simulink model "VHF_central_unit"  (R2024a)
settings: Solver=FixedStepDiscrete  StartTime=0.0  StopTime=10.0  FixedStep=0.001  RelTol=1e-3  EnableMultiTasking=on
PreLoadFcn:
  | try
  | MDL_install;
  | catch
  | end
InitFcn:
  | EcoCoder_PreCheckLic();
undefined symbols (not defined in the file or in its folder): C_ROTSPD_ZERO, C_SOC_ZERO, h, km, s, V
libraries: CoderSF_BSW_Libs x222, SF_CanService_Libs x16, CoderSF_ADC2Volt_Libs x6, CoderSF_6AxisMEMS_Libs x6, canmsglib x3, EV_ASWLibs x2, simulink x2, Chassis_stability_controllers x1, CoderSF_KeyCycle_Libs x1
(part 3 of 4)

== system VHF_central_unit/ASW_ReadCAN/Read BMS messages/Subsystem ==
  In1 : Inport
  Bus Creator1 : BusCreator  Inputs=4
  Bus Creator2 : BusCreator  Inputs=4
  Bus Selector : BusSelector  OutputSignals=BMS_OperationStatus.BMSBattPackVoltage,BMS_OperationStatus.BMSBattOCV,BMS_OperationStatus.BMSBattPackCurrent,BMS_OperationStatus.BMSPackMaxDischargeCurrent,BMS_OperationStatus.BMSPackMaxChargeCurrent,BMS_StateOfStatus.BMSStateOfCharge,BMS_StateOfStatus.BMSStateOfHealth,BMS_StateOfStatus.BMSStateOfEnergy,BMS_StateOfStatus.BMSBattStoragedEnergy,BMS_StateOfStatus.BMSBattTemperature,BMS_CellVoltage1to8.BMSCellVoltage1,BMS_CellVoltage1to8.BMSCellVoltage2,BMS_CellVoltage1to8.BMSCellVoltage3,BMS_CellVoltage1to8.BMSCellVoltage4,BMS_CellVoltage1to8.BMSCellVoltage5,BMS_CellVoltage1to8.BMSCellVoltage6,BMS_CellVoltage1to8.BMSCellVoltage7,BMS_CellVoltage1to8.BMSCellVoltage8,BMS_CellVoltage9to16.BMSCellVoltage9,BMS_CellVoltage9to16.BMSCellVoltage10,BMS_CellVoltage9to16.BMSCellVoltage11,BMS_CellVoltage9to16.BMSCellVoltage12,BMS_CellVoltage9to16.BMSCellVoltage13,BMS_CellVoltage9to16.BMSCellVoltage14,BMS_CellVoltage9to16.BMSCellVoltage15,BMS_CellVoltage9to16.BMSCellVoltage16  OutputAsBus=on
  Bus Selector1 : BusSelector  OutputSignals=BMS_OperationStatus.signal1,BMS_StateOfStatus.signal1,BMS_CellVoltage1to8.signal1,BMS_CellVoltage9to16.signal1
  Bus Selector2 : BusSelector  OutputSignals=BMS_OperationStatus.signal2,BMS_StateOfStatus.signal2,BMS_CellVoltage1to8.signal2,BMS_CellVoltage9to16.signal2
  Data Type Conversion{,1..7} (8 alike) : DataTypeConversion  SaturateOnIntegerOverflow=off  RndMeth=Floor
  BMSmsgs : Outport
  MsgAvailable : Outport  Port=2
  MsgCount : Outport  Port=3
  wires:
  Bus Selector/1 -> BMSmsgs/1  "BMSmsgs"
  Bus Selector1/1 -> Data Type Conversion/1  "<signal1>"
  Bus Selector1/2 -> Data Type Conversion1/1  "<signal1>"
  Bus Selector1/3 -> Data Type Conversion2/1  "<signal1>"
  Bus Selector1/4 -> Data Type Conversion3/1  "<signal1>"
  Data Type Conversion/1 -> Bus Creator1/1  "MsgAvailable_OperationStatus"
  Data Type Conversion1/1 -> Bus Creator1/2  "MsgAvailable_StateOfStatus"
  Data Type Conversion2/1 -> Bus Creator1/3  "MsgAvailable_CellVoltage1to8"
  Data Type Conversion3/1 -> Bus Creator1/4  "MsgAvailable_CellVoltage9to16"
  Data Type Conversion7/1 -> Bus Creator2/4  "MsgCount_CellVoltage9to16"
  Data Type Conversion4/1 -> Bus Creator2/1  "MsgCount_OperationStatus"
  Bus Selector2/3 -> Data Type Conversion6/1  "<signal2>"
  Data Type Conversion6/1 -> Bus Creator2/3  "MsgCount_CellVoltage1to8"
  Bus Selector2/2 -> Data Type Conversion5/1  "<signal2>"
  Bus Selector2/4 -> Data Type Conversion7/1  "<signal2>"
  Data Type Conversion5/1 -> Bus Creator2/2  "MsgCount_StateOfStatus"
  Bus Selector2/1 -> Data Type Conversion4/1  "<signal2>"
  In1/1 -> Bus Selector2/1, Bus Selector1/1, Bus Selector/1
  Bus Creator1/1 -> MsgAvailable/1  "MsgAvailable"
  Bus Creator2/1 -> MsgCount/1  "MsgCount"

== system VHF_central_unit/ASW_ReadCAN/Read CCU messages/Subsystem ==
  In1 : Inport
  Bus Creator1 : BusCreator  Inputs=2
  Bus Creator2 : BusCreator  Inputs=2
  Bus Selector : BusSelector  OutputSignals=CCU_Status_VCU.CCUDccOutVoltage,CCU_Status_VCU.CCUDccOutCurrent,CCU_Status_VCU.CCUInputCurrent,CCU_Status_VCU.CCUControlMode,CCU_Status_VCU.CCURegenerateMode,CCU_Status_VCU.CCUFaultControl,CCU_Status_VCU.CCUUnderBattVolt,CCU_Status_VCU.CCUOverBattVolt,CCU_Status_VCU.CCUOverInd1Curr,CCU_Status_VCU.CCUOverInd2Curr,CCU_Status_VCU.CCUOverInd3Curr,CCU_Status_VCU.CCULeg1Failure,CCU_Status_VCU.CCULeg2Failure,CCU_Status_VCU.CCULeg3Failure,CCU_Status_VCU.CCUOverOutVolt,CCU_InductorStatus.CCUInductor1Curr,CCU_InductorStatus.CCUInductor2Curr,CCU_InductorStatus.CCUInductor3Curr  OutputAsBus=on
  Bus Selector1 : BusSelector  OutputSignals=CCU_Status_VCU.signal1,CCU_InductorStatus.signal1
  Bus Selector2 : BusSelector  OutputSignals=CCU_Status_VCU.signal2,CCU_InductorStatus.signal2
  Data Type Conversion{,1,4..5} (4 alike) : DataTypeConversion  SaturateOnIntegerOverflow=off  RndMeth=Floor
  CCUmsgs : Outport
  MsgAvailable : Outport  Port=2
  MsgCount : Outport  Port=3
  wires:
  Bus Selector/1 -> CCUmsgs/1  "CCUmsgs"
  Bus Selector1/1 -> Data Type Conversion/1  "<signal1>"
  Bus Selector1/2 -> Data Type Conversion1/1  "<signal1>"
  Data Type Conversion/1 -> Bus Creator1/1  "MsgAvailable_CCU_Status_VCU"
  Data Type Conversion1/1 -> Bus Creator1/2  "MsgAvailable_CCU_InductorStatus"
  Data Type Conversion4/1 -> Bus Creator2/1  "MsgCount_CCU_Status_VCU"
  Bus Selector2/2 -> Data Type Conversion5/1  "<signal2>"
  Data Type Conversion5/1 -> Bus Creator2/2  "MsgCount_CCU_InductorStatus"
  Bus Selector2/1 -> Data Type Conversion4/1  "<signal2>"
  In1/1 -> Bus Selector2/1, Bus Selector1/1, Bus Selector/1
  Bus Creator1/1 -> MsgAvailable/1  "MsgAvailable"
  Bus Creator2/1 -> MsgCount/1  "MsgCount"

== system VHF_central_unit/ASW_ReadCAN/Read GeneratorSystem messages/Subsystem ==
  In1 : Inport
  Bus Creator1 : BusCreator  Inputs=2
  Bus Creator2 : BusCreator  Inputs=2
  Bus Selector : BusSelector  OutputSignals=SCG_Status_VCU.GenSysDccOutVoltage,SCG_Status_VCU.GenSysDccOutCurrent,SCG_Status_VCU.GenSysGenVoltage,SCG_Status_VCU.GenSysGenCurrent,SCG_Status_VCU.GenSysControlMode,SCG_Status_VCU.GenSysAcRelayStatus,SCG_Status_VCU.GenSysLinkPosRelay,SCG_Status_VCU.GenSysFaultControl,SCG_Status_VCU.GenSysOverOutVolt,SCG_Status_VCU.GenSysOverInd1Curr,SCG_Status_VCU.GenSysOverInd2Curr,SCG_Status_VCU.GenSysOverInd3Curr,SCG_Status_VCU.GenSysLeg1Failure,SCG_Status_VCU.GenSysLeg2Failure,SCG_Status_VCU.GenSysLeg3Failure,SCG_ICE_Status.GenSysMotorTorque,SCG_ICE_Status.GenSysMotorSpeed,SCG_ICE_Status.GenSysThrottle  OutputAsBus=on
  Bus Selector1 : BusSelector  OutputSignals=SCG_Status_VCU.signal1,SCG_ICE_Status.signal1
  Bus Selector2 : BusSelector  OutputSignals=SCG_Status_VCU.signal2,SCG_ICE_Status.signal2
  Data Type Conversion{,1,4..5} (4 alike) : DataTypeConversion  SaturateOnIntegerOverflow=off  RndMeth=Floor
  SCGmsgs : Outport
  MsgAvailable : Outport  Port=2
  MsgCount : Outport  Port=3
  wires:
  Bus Selector/1 -> SCGmsgs/1  "SCGmsgs"
  Bus Selector1/1 -> Data Type Conversion/1  "<signal1>"
  Bus Selector1/2 -> Data Type Conversion1/1  "<signal1>"
  Data Type Conversion/1 -> Bus Creator1/1  "MsgAvailable_SCG_Status_VCU"
  Data Type Conversion1/1 -> Bus Creator1/2  "MsgAvailable_SCG_ICE_Status"
  Data Type Conversion4/1 -> Bus Creator2/1  "MsgCount_SCG_Status_VCU"
  Bus Selector2/2 -> Data Type Conversion5/1  "<signal2>"
  Data Type Conversion5/1 -> Bus Creator2/2  "MsgCount_SCG_ICE_Status"
  Bus Selector2/1 -> Data Type Conversion4/1  "<signal2>"
  In1/1 -> Bus Selector2/1, Bus Selector1/1, Bus Selector/1
  Bus Creator1/1 -> MsgAvailable/1  "MsgAvailable"
  Bus Creator2/1 -> MsgCount/1  "MsgCount"

== system VHF_central_unit/ASW_ReadCAN/Read Motor1 messages/Subsystem ==
  In1 : Inport
  Bus Creator1 : BusCreator  Inputs=2
  Bus Creator2 : BusCreator  Inputs=2
  Bus Selector : BusSelector  OutputSignals=Motor1_RUN_STATUS.Motor1Run_direction,Motor1_RUN_STATUS.Motor1Running_mode,Motor1_RUN_STATUS.Motor1Motor_Speed,Motor1_RUN_STATUS.Motor1Fault_Code,Motor1_RUN_STATUS.Motor1ConsumptionMode,Motor1_RUN_STATUS.Motor1SubtotalMileage,Motor1_ELEC_STATUS.Motor1DC_LinkVoltage,Motor1_ELEC_STATUS.Motor1DC_LinkCurrent  OutputAsBus=on
  Bus Selector1 : BusSelector  OutputSignals=Motor1_RUN_STATUS.signal1,Motor1_ELEC_STATUS.signal1
  Bus Selector2 : BusSelector  OutputSignals=Motor1_RUN_STATUS.signal2,Motor1_ELEC_STATUS.signal2
  Data Type Conversion{,1,4..5} (4 alike) : DataTypeConversion  SaturateOnIntegerOverflow=off  RndMeth=Floor
  Motor1msgs : Outport
  MsgAvailable : Outport  Port=2
  MsgCount : Outport  Port=3
  wires:
  Bus Selector/1 -> Motor1msgs/1  "Motor1msgs"
  Bus Selector1/1 -> Data Type Conversion/1  "<signal1>"
  Bus Selector1/2 -> Data Type Conversion1/1  "<signal1>"
  Data Type Conversion/1 -> Bus Creator1/1  "MsgAvailable_RUN_STATUS"
  Data Type Conversion1/1 -> Bus Creator1/2  "MsgAvailable_ELEC_STATUS"
  Data Type Conversion4/1 -> Bus Creator2/1  "MsgCount_RUN_STATUS"
  Bus Selector2/2 -> Data Type Conversion5/1  "<signal2>"
  Data Type Conversion5/1 -> Bus Creator2/2  "MsgCount_ELEC_STATUS"
  Bus Selector2/1 -> Data Type Conversion4/1  "<signal2>"
  In1/1 -> Bus Selector2/1, Bus Selector1/1, Bus Selector/1
  Bus Creator1/1 -> MsgAvailable/1  "MsgAvailable"
  Bus Creator2/1 -> MsgCount/1  "MsgCount"

== system VHF_central_unit/ASW_ReadCAN/Read Motor2 messages/Subsystem ==
  In1 : Inport
  Bus Creator1 : BusCreator  Inputs=2
  Bus Creator2 : BusCreator  Inputs=2
  Bus Selector : BusSelector  OutputSignals=Motor2_RUN_STATUS.Motor2Run_direction,Motor2_RUN_STATUS.Motor2Running_mode,Motor2_RUN_STATUS.Motor2Motor_Speed,Motor2_RUN_STATUS.Motor2Fault_Code,Motor2_RUN_STATUS.Motor2ConsumptionMode,Motor2_RUN_STATUS.Motor2SubtotalMileage,Motor2_ELEC_STATUS.Motor2DC_LinkVoltage,Motor2_ELEC_STATUS.Motor2DC_LinkCurrent  OutputAsBus=on
  Bus Selector1 : BusSelector  OutputSignals=Motor2_RUN_STATUS.signal1,Motor2_ELEC_STATUS.signal1
  Bus Selector2 : BusSelector  OutputSignals=Motor2_RUN_STATUS.signal2,Motor2_ELEC_STATUS.signal2
  Data Type Conversion{,1,4..5} (4 alike) : DataTypeConversion  SaturateOnIntegerOverflow=off  RndMeth=Floor
  Motor2msgs : Outport
  MsgAvailable : Outport  Port=2
  MsgCount : Outport  Port=3
  wires:
  Bus Selector/1 -> Motor2msgs/1  "Motor2msgs"
  Bus Selector1/1 -> Data Type Conversion/1  "<signal1>"
  Bus Selector1/2 -> Data Type Conversion1/1  "<signal1>"
  Data Type Conversion/1 -> Bus Creator1/1  "MsgAvailable_RUN_STATUS"
  Data Type Conversion1/1 -> Bus Creator1/2  "MsgAvailable_ELEC_STATUS"
  Data Type Conversion4/1 -> Bus Creator2/1  "MsgCount_RUN_STATUS"
  Bus Selector2/2 -> Data Type Conversion5/1  "<signal2>"
  Data Type Conversion5/1 -> Bus Creator2/2  "MsgCount_ELEC_STATUS"
  Bus Selector2/1 -> Data Type Conversion4/1  "<signal2>"
  In1/1 -> Bus Selector2/1, Bus Selector1/1, Bus Selector/1
  Bus Creator1/1 -> MsgAvailable/1  "MsgAvailable"
  Bus Creator2/1 -> MsgCount/1  "MsgCount"

== system VHF_central_unit/ASW_SensorInputs/02 vehicle motion request/01 driver torque demand ==
  sigInDrvPedacc_pct1 : Inport
  f : TriggerPort  TriggerType=function-call  VariantControl=(inherit)
  Switch : Switch  Criteria=u2 ~= 0  SaturateOnIntegerOverflow=off  InputSameDT=off
  ecocoder_calibration : CoderSF_BSW_Libs/Calibration & Measurement/Read Calibration  variable_name=vehDrv_flgCal_val  variable_value=0  variable_type=boolean  variable_min=[]  variable_max=[]  unitStr=""  descStr=""
      settings: AttributesFormatString=value:%<variable_value> type:%<variable_type> max:%<variable_max> Min:%<variable_min>
  ecocoder_calibration1 : CoderSF_BSW_Libs/Calibration & Measurement/Read Calibration  variable_name=vehDrv_linspd_val  variable_value=0  variable_type=single  variable_min=[]  variable_max=[]  unitStr=km/h  descStr=""
      settings: AttributesFormatString=value:%<variable_value> type:%<variable_type> max:%<variable_max> Min:%<variable_min>
  ecocoder_calibration2 : CoderSF_BSW_Libs/Calibration & Measurement/Read Calibration  variable_name=vehDrv_pct_val  variable_value=0  variable_type=single  variable_min=[]  variable_max=[]  unitStr=""  descStr=""
      settings: AttributesFormatString=value:%<variable_value> type:%<variable_type> max:%<variable_max> Min:%<variable_min>
  ecocoder_measurement : CoderSF_BSW_Libs/Calibration & Measurement/Write and Read Measurement  variable_name=vehDrv_linspd  variable_value=0  variable_type=single  numD=1  unitStr=km/h  descStr=""
      settings: AttributesFormatString=value:%<variable_value> type:%<variable_type>
  ecocoder_measurement1 : CoderSF_BSW_Libs/Calibration & Measurement/Write and Read Measurement  variable_name=vehDrv_pct  variable_value=0  variable_type=single  numD=1  unitStr=""  descStr=""
      settings: AttributesFormatString=value:%<variable_value> type:%<variable_type>
  ecocoder_measurement2 : CoderSF_BSW_Libs/Calibration & Measurement/Write and Read Measurement  variable_name=vehDrv_trqReq  variable_value=0  variable_type=single  numD=1  unitStr=Nm  descStr=""
      settings: AttributesFormatString=value:%<variable_value> type:%<variable_type>
  vehDrv_trqEcoTracMax_map : CoderSF_BSW_Libs/Calibration & Measurement/2-D Lookup Table  nam=vehDrv_trqEcoTracMax  breakpoint1_type=single  breakpoint1_data=[0 0.1 0.2 0.3 0.4 0.5 0.6 0.7 0.8 0.9 0.95 1]  breakpoint2_type=single  breakpoint2_data="[0 2 3 10  20 30 40 50 60 70 80 90 95 100 115 120]"  table_type=single  table_data=|
      | [0 0 0 0 0 0 0 0 0 0 0 0 0 0 0 0 ;
      | 0 200 441 439 437 435 433 431 429 427 425 423 421 419 417 415 ;
      | 0 202 461 459 457 455 453 451 449 447 445 443 441 439 437 435 ;
      | 0 204 565 560 555 550 545 540 535 530 525 520 515 510 505 500 ;
      | 0 206 614 611 608 605 602 599 596 593 590 587 584 581 578 575 ;
      | 0 208 678 677 676 675 674 673 672 671 670 669 668 667 666 665 ;
      | 0 210 784 781 778 775 772 769 766 763 760 757 754 751 748 745 ;
      | 0 212 956 954 952 950 948 946 944 942 940 938 936 934 932 930 ;
      | 0 214 1078 1077 1076 1075 1074 1073 1072 1071 1070 1069 1068 1067 1066 1065 ;
      | 0 216 1376 1374 1372 1370 1368 1366 1364 1362 1360 1358 1356 1354 1352 1350 ;
      | 0 218 1576 1574 1572 1570 1568 1566 1564 1562 1560 1558 1556 1554 1552 1550 ;
      | 0 220 1900 1900 1900 1900 1900 1900 1900 1900 1900 1900 1900 1900 1900 1900 ]
  vehDrv_trqReq1 : Outport
  wires:
  vehDrv_trqEcoTracMax_map/1 -> ecocoder_measurement2/1
  ecocoder_calibration1/1 -> ecocoder_measurement/1
  sigInDrvPedacc_pct1/1 -> Switch/3
  Switch/1 -> ecocoder_measurement1/1
  ecocoder_calibration/1 -> Switch/2
  ecocoder_calibration2/1 -> Switch/1
  ecocoder_measurement/1 -> vehDrv_trqEcoTracMax_map/2  "vehDrv_linspd"
  ecocoder_measurement1/1 -> vehDrv_trqEcoTracMax_map/1  "vehDrv_pct"
  ecocoder_measurement2/1 -> vehDrv_trqReq1/1  "vehDrv_trqReq"

== system VHF_central_unit/ASW_SensorInputs/Accelerator read/Accelerator In ==
  function : TriggerPort  TriggerType=function-call  VariantControl=(inherit)
  ADC Value To Volt : CoderSF_ADC2Volt_Libs/ADC Value To Volt  ResValue=12  RefValue=5  TypeOut=single  WithDiv=off  DivValue=16  SerValue=100
  Gain : Gain  Gain=1/5
  Read ADC Value : CoderSF_BSW_Libs/ADC/Read ADC Value  channel=3
  Read Calibration : CoderSF_BSW_Libs/Calibration & Measurement/Read Calibration  variable_name=AccInputAnalogMax  variable_value=4.9  variable_type=single  variable_min=[]  variable_max=[]  unitStr=V  descStr=Upper limit of the analog signal from accelerator
      settings: AttributesFormatString=value:%<variable_value> type:%<variable_type> max:%<variable_max> Min:%<variable_min>
  Read Calibration1 : CoderSF_BSW_Libs/Calibration & Measurement/Read Calibration  variable_name=AccInputAnalogMin  variable_value=0.1  variable_type=single  variable_min=[]  variable_max=[]  unitStr=V  descStr=Lower limit of the analog signal from accelerator
      settings: AttributesFormatString=value:%<variable_value> type:%<variable_type> max:%<variable_max> Min:%<variable_min>
  Saturation Dynamic : simulink/Discontinuities/Saturation Dynamic  OutMin=[]  OutMax=[]  OutDataTypeStr=Inherit: Same as second input  OutDataType=fixdt(1, 16)  OutScaling=2^-10  DoSatur=off
  Write and Read Measurement : CoderSF_BSW_Libs/Calibration & Measurement/Write and Read Measurement  variable_name=AccInputVar  variable_value=0  variable_type=single  numD=1  unitStr=V  descStr=Analog Input of the accelerator pedal
      settings: AttributesFormatString=type:%<variable_type> Dimensions:%<numD>
  thrtl : Outport
  wires:
  ADC Value To Volt/1 -> Saturation Dynamic/2
  Read ADC Value/1 -> Write and Read Measurement/1
  Write and Read Measurement/1 -> ADC Value To Volt/1  "AccInputVar"
  Saturation Dynamic/1 -> Gain/1
  Gain/1 -> thrtl/1
  Read Calibration/1 -> Saturation Dynamic/1
  Read Calibration1/1 -> Saturation Dynamic/3

== system VHF_central_unit/ASW_SensorInputs/Brake read/Get Brake signal ==
  function : TriggerPort  TriggerType=function-call  VariantControl=(inherit)
  ADC Value To Volt : CoderSF_ADC2Volt_Libs/ADC Value To Volt  ResValue=12  RefValue=5  TypeOut=single  WithDiv=off  DivValue=16  SerValue=100
  Hysteresis : CoderSF_BSW_Libs/Application Base Blocks/Hysteresis
  Read ADC Value : CoderSF_BSW_Libs/ADC/Read ADC Value  channel=1
  Read Calibration : CoderSF_BSW_Libs/Calibration & Measurement/Read Calibration  variable_name=BrkInMaxThrs  variable_value=1  variable_type=single  variable_min=[]  variable_max=[]  unitStr=V  descStr=Maximum Threshhold for brake signal
      settings: AttributesFormatString=value:%<variable_value> type:%<variable_type> max:%<variable_max> Min:%<variable_min>
  Read Calibration2 : CoderSF_BSW_Libs/Calibration & Measurement/Read Calibration  variable_name=BrkInMixThrs  variable_value=0.5  variable_type=single  variable_min=[]  variable_max=[]  unitStr=V  descStr=Minimum Threshhold for brake signal
      settings: AttributesFormatString=value:%<variable_value> type:%<variable_type> max:%<variable_max> Min:%<variable_min>
  Write and Read Measurement : CoderSF_BSW_Libs/Calibration & Measurement/Write and Read Measurement  variable_name=AccInputVar  variable_value=0  variable_type=single  numD=1  unitStr=V  descStr=Analog Input of the accelerator pedal
      settings: AttributesFormatString=type:%<variable_type> Dimensions:%<numD>
  brk : Outport
  wires:
  Hysteresis/1 -> brk/1
  ADC Value To Volt/1 -> Hysteresis/2
  Read Calibration/1 -> Hysteresis/1
  Read Calibration2/1 -> Hysteresis/3
  Read ADC Value/1 -> Write and Read Measurement/1
  Write and Read Measurement/1 -> ADC Value To Volt/1  "AccInputVar"

== system VHF_central_unit/ASW_SensorInputs/MEMS sensor read/Estimate speed ==
  Accel : Inport
  Gyro : Inport  Port=2
  function : TriggerPort  TriggerType=function-call  VariantControl=(inherit)
  Vspeed : Outport
  Orientation : Outport  Port=2

== system VHF_central_unit/ASW_SensorInputs/MEMS sensor read/Read Sensor Data ==
  function : TriggerPort  TriggerType=function-call  VariantControl=(inherit)
  Constant : Constant  OutDataTypeStr=Inherit: Inherit via back propagation  SampleTime=-1
  "Read Fixed NVM " : CoderSF_BSW_Libs/Non-volatile Memory Blocks/Read Fixed NVM   data_name=Fnvm_Sensor_stSelfTest
  Relational Operator : RelationalOperator  Operator===  OutDataTypeStr=boolean  InputSameDT=off
  Subsystem : Subsystem
  ID : Outport
  Accel : Outport  Port=2
  Gyro : Outport  Port=3
  Temp : Outport  Port=4
  wires:
  "Read Fixed NVM "/1 -> Relational Operator/1
  Constant/1 -> Relational Operator/2
  Relational Operator/1 -> Subsystem/Enable
  Subsystem/1(ID) -> ID/1
  Subsystem/2(Accel) -> Accel/1
  Subsystem/3(Gyro) -> Gyro/1
  Subsystem/4(Temp) -> Temp/1

== system VHF_central_unit/ASW_SensorInputs/Read BMS msgs/Subsystem1 ==
  function : TriggerPort  TriggerType=function-call  VariantControl=(inherit)
  Constant : Constant
  Out1 : Outport
  wires:
  Constant/1 -> Out1/1

== system VHF_central_unit/ASW_SensorInputs/Read DCDC converter msgs/Subsystem1 ==
  function : TriggerPort  TriggerType=function-call  VariantControl=(inherit)
  Constant : Constant
  Out1 : Outport
  wires:
  Constant/1 -> Out1/1

== system VHF_central_unit/ASW_SensorInputs/Read GenSys msgs/Subsystem1 ==
  function : TriggerPort  TriggerType=function-call  VariantControl=(inherit)
  Constant : Constant
  Out1 : Outport
  wires:
  Constant/1 -> Out1/1

== system VHF_central_unit/ASW_SensorInputs/Read Inverter 1/Subsystem1 ==
  function : TriggerPort  TriggerType=function-call  VariantControl=(inherit)
  Constant : Constant
  Out1 : Outport
  wires:
  Constant/1 -> Out1/1

== system VHF_central_unit/ASW_SensorInputs/Read Inverter 2/Subsystem1 ==
  function : TriggerPort  TriggerType=function-call  VariantControl=(inherit)
  Constant : Constant
  Out1 : Outport
  wires:
  Constant/1 -> Out1/1

== system VHF_central_unit/ASW_Demo/01  process input signals/01 process electrical supply input signals/02 process electrical supply input signals ==
  f : TriggerPort  TriggerType=function-call  VariantControl=(inherit)
  01 process battery voltage : Subsystem  TreatAsAtomicUnit=on
      settings: RTWSystemCode=Nonreusable function
  sigInEsmBatt_volt : Outport
  wires:
  01 process battery voltage/1(sigInEsmBatt_volt) -> sigInEsmBatt_volt/1

== system VHF_central_unit/ASW_Demo/01  process input signals/02 process driver input signals/01 link driver input signals ==
  f : TriggerPort  TriggerType=function-call  VariantControl=(inherit)
  01 link key position : Subsystem
  03 link accelerator pedal : Subsystem
  sigInLinkDrvKey_flgOn : Outport
  sigInLinkDrvPedacc_volt1 : Outport  Port=2
  sigInLinkDrvPedacc_volt2 : Outport  Port=3
  wires:
  03 link accelerator pedal/2(sigInLinkDrvPedacc_volt2) -> sigInLinkDrvPedacc_volt2/1
  03 link accelerator pedal/1(sigInLinkDrvPedacc_volt1) -> sigInLinkDrvPedacc_volt1/1
  01 link key position/1(sigInLinkDrvKey_flgOn) -> sigInLinkDrvKey_flgOn/1

== system VHF_central_unit/ASW_Demo/01  process input signals/02 process driver input signals/02 process driver input signals ==
  sigInLinkDrvPedacc_volt1 : Inport
  sigInLinkDrvPedacc_volt2 : Inport  Port=2
  f : TriggerPort  TriggerType=function-call  VariantControl=(inherit)
  03 processs accelerator pedal : Subsystem
  sigInDrvPedacc_pct : Outport
  wires:
  sigInLinkDrvPedacc_volt1/1 -> 03 processs accelerator pedal/1(sigInLinkDrvPedacc_volt1)
  sigInLinkDrvPedacc_volt2/1 -> 03 processs accelerator pedal/2(sigInLinkDrvPedacc_volt2)
  03 processs accelerator pedal/1(sigInDrvPedacc_pct) -> sigInDrvPedacc_pct/1

== system VHF_central_unit/ASW_Demo/01  process input signals/03 process bms input signals/00 process bms input signals ==
  sigInBms_socRaw : Inport
  f : TriggerPort  TriggerType=function-call  VariantControl=(inherit)
  02 process bms soc : Subsystem  TreatAsAtomicUnit=on
      settings: RTWSystemCode=Nonreusable function
  Constant : Constant  Value=true  SampleTime=-1
  sigInBms_soc : Outport
  wires:
  Constant/1 -> 02 process bms soc/2(sigInBms_flgSocRawValid)
  sigInBms_socRaw/1 -> 02 process bms soc/1(sigInBms_socRaw)
  02 process bms soc/1(sigInBms_soc) -> sigInBms_soc/1

== system VHF_central_unit/ASW_Demo/01  process input signals/04 process traction motor input signals/00 process traction motor input signals ==
  sigInMot_rotspdRpm : Inport
  sigInMot_flgRotspdRpmValid : Inport  Port=2
  f : TriggerPort  TriggerType=function-call  VariantControl=(inherit)
  02 motor speed calculation : Subsystem  TreatAsAtomicUnit=on
      settings: RTWSystemCode=Nonreusable function
  sigInTm_rotspd : Outport
  wires:
  sigInMot_flgRotspdRpmValid/1 -> 02 motor speed calculation/2(sigInMot_flgRotspdRpmValid)
  sigInMot_rotspdRpm/1 -> 02 motor speed calculation/1(sigInMot_rotspdRpm)
  02 motor speed calculation/1(sigInTm_rotspd) -> sigInTm_rotspd/1

== system VHF_central_unit/ASW_Demo/03 electrical supply management/02  electrical supply control/esmc ==
  sigInEsmBatt_volt : Inport
  f : TriggerPort  TriggerType=function-call  VariantControl=(inherit)
  Constant : Constant  OutDataTypeStr=Inherit: Inherit via back propagation  SampleTime=-1
  Terminator : Terminator
  esmcDcdc_flgEn : Outport
  wires:
  Constant/1 -> esmcDcdc_flgEn/1  "esmcDcdc_flgEn"
  sigInEsmBatt_volt/1 -> Terminator/1

== system VHF_central_unit/ASW_Demo/04 powertrain control /02  Bms control/02  Bms control ==
  pwrtrn_stVeh : Inport
  Task_Call4 : CoderSF_BSW_Libs/Task Scheduler/Task Trigger  tasktimeIndex=Task_L20ms
  bmsc : Subsystem  TreatAsAtomicUnit=on
  pwrtrnBmscPack_flgConnReq : Outport
  wires:
  bmsc/1(pwrtrnBmscPack_flgConnReq) -> pwrtrnBmscPack_flgConnReq/1
  Task_Call4/1 -> bmsc/Trigger
  pwrtrn_stVeh/1 -> bmsc/1(pwrtrn_st_i)

== system VHF_central_unit/ASW_Demo/04 powertrain control /03  traction motor control/tmc ==
  sigInTm_rotspd : Inport
  vehDrv_trqReq : Inport  Port=2
  f : TriggerPort  TriggerType=function-call  VariantControl=(inherit)
  02 torque calculation : Subsystem
  Constant : Constant  Value=2  OutDataTypeStr=Inherit: Inherit via back propagation
  pwrtrnTmc_trqCmd : Outport
  wires:
  Constant/1 -> 02 torque calculation/2(pwrtrnTml_ratioShaftRotspd)  "pwrtrnTml_ratioShaftRotspd"
  sigInTm_rotspd/1 -> 02 torque calculation/3(sigInTm_rotspd)
  vehDrv_trqReq/1 -> 02 torque calculation/1(vehDrv_trqReq)
  02 torque calculation/1(pwrtrnTmc_trqReq) -> pwrtrnTmc_trqCmd/1

== system VHF_central_unit/ASW_Demo/06 process output signals/01 process electrical supply output signals/01 process electrical supply output signals ==
  esmcDcdc_flgEn : Inport
  f : TriggerPort  TriggerType=function-call  VariantControl=(inherit)
  Terminator : Terminator
  wires:
  esmcDcdc_flgEn/1 -> Terminator/1

== system VHF_central_unit/ASW_Demo/06 process output signals/02 process traction motor output signals/02 process traction motor output signals ==
  pwrtrnTmc_trqCmd : Inport  Interpolate=off
  f : TriggerPort  TriggerType=function-call  VariantControl=(inherit)
  DT_conv5 : DataTypeConversion  SaturateOnIntegerOverflow=off  RndMeth=Floor
  txMCU_trqReq : Outport
  wires:
  DT_conv5/1 -> txMCU_trqReq/1  "txMCU_trqReq"
  pwrtrnTmc_trqCmd/1 -> DT_conv5/1

== system VHF_central_unit/ASW_Demo/06 process output signals/03 process bms output signals/03 process bms output signals ==
  pwrtrnBmscPack_flgConnReq : Inport
  f : TriggerPort  TriggerType=function-call  VariantControl=(inherit)
  DT_conv1 : DataTypeConversion  SaturateOnIntegerOverflow=off  RndMeth=Floor
  sigOutBms_flgConnHv : Outport
  wires:
  DT_conv1/1 -> sigOutBms_flgConnHv/1  "txBMS_stPwrCmd"
  pwrtrnBmscPack_flgConnReq/1 -> DT_conv1/1

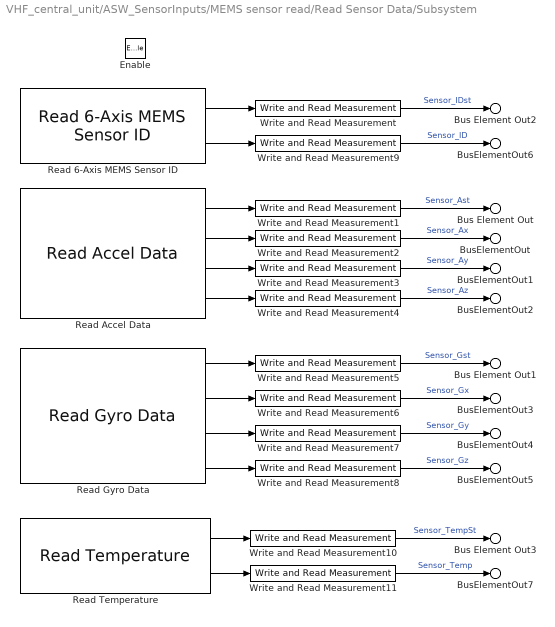
== system VHF_central_unit/ASW_SensorInputs/MEMS sensor read/Read Sensor Data/Subsystem ==
  Enable : EnablePort
  Read 6-Axis MEMS Sensor ID : CoderSF_6AxisMEMS_Libs/6-Axis MEMS Sensor/Read 6-Axis MEMS Sensor ID
  Read Accel Data : CoderSF_6AxisMEMS_Libs/6-Axis MEMS Sensor/Read Accel Data
  Read Gyro Data : CoderSF_6AxisMEMS_Libs/6-Axis MEMS Sensor/Read Gyro Data
  Read Temperature : CoderSF_6AxisMEMS_Libs/6-Axis MEMS Sensor/Read Temperature
  Write and Read Measurement : CoderSF_BSW_Libs/Calibration & Measurement/Write and Read Measurement  variable_name=Sensor_IDst  variable_value=0  variable_type=uint8  numD=1  unitStr=""  descStr=""
      settings: AttributesFormatString=type:%<variable_type> Dimensions:%<numD>
  Write and Read Measurement1 : CoderSF_BSW_Libs/Calibration & Measurement/Write and Read Measurement  variable_name=Sensor_Ast  variable_value=0  variable_type=uint8  numD=1  unitStr=""  descStr=""
      settings: AttributesFormatString=type:%<variable_type> Dimensions:%<numD>
  Write and Read Measurement10 : CoderSF_BSW_Libs/Calibration & Measurement/Write and Read Measurement  variable_name=Sensor_TempSt  variable_value=0  variable_type=uint8  numD=1  unitStr=""  descStr=""
      settings: AttributesFormatString=type:%<variable_type> Dimensions:%<numD>
  Write and Read Measurement11 : CoderSF_BSW_Libs/Calibration & Measurement/Write and Read Measurement  variable_name=Sensor_Temp  variable_value=0  variable_type=single  numD=1  unitStr=""  descStr=""
      settings: AttributesFormatString=type:%<variable_type> Dimensions:%<numD>
  Write and Read Measurement2 : CoderSF_BSW_Libs/Calibration & Measurement/Write and Read Measurement  variable_name=Sensor_Ax  variable_value=0  variable_type=int16  numD=1  unitStr=""  descStr=""
      settings: AttributesFormatString=type:%<variable_type> Dimensions:%<numD>
  Write and Read Measurement3 : CoderSF_BSW_Libs/Calibration & Measurement/Write and Read Measurement  variable_name=Sensor_Ay  variable_value=0  variable_type=int16  numD=1  unitStr=""  descStr=""
      settings: AttributesFormatString=type:%<variable_type> Dimensions:%<numD>
  Write and Read Measurement4 : CoderSF_BSW_Libs/Calibration & Measurement/Write and Read Measurement  variable_name=Sensor_Az  variable_value=0  variable_type=int16  numD=1  unitStr=""  descStr=""
      settings: AttributesFormatString=type:%<variable_type> Dimensions:%<numD>
  Write and Read Measurement5 : CoderSF_BSW_Libs/Calibration & Measurement/Write and Read Measurement  variable_name=Sensor_Gst  variable_value=0  variable_type=uint8  numD=1  unitStr=""  descStr=""
      settings: AttributesFormatString=type:%<variable_type> Dimensions:%<numD>
  Write and Read Measurement6 : CoderSF_BSW_Libs/Calibration & Measurement/Write and Read Measurement  variable_name=Sensor_Gx  variable_value=0  variable_type=int16  numD=1  unitStr=""  descStr=""
      settings: AttributesFormatString=type:%<variable_type> Dimensions:%<numD>
  Write and Read Measurement7 : CoderSF_BSW_Libs/Calibration & Measurement/Write and Read Measurement  variable_name=Sensor_Gy  variable_value=0  variable_type=int16  numD=1  unitStr=""  descStr=""
      settings: AttributesFormatString=type:%<variable_type> Dimensions:%<numD>
  Write and Read Measurement8 : CoderSF_BSW_Libs/Calibration & Measurement/Write and Read Measurement  variable_name=Sensor_Gz  variable_value=0  variable_type=int16  numD=1  unitStr=""  descStr=""
      settings: AttributesFormatString=type:%<variable_type> Dimensions:%<numD>
  Write and Read Measurement9 : CoderSF_BSW_Libs/Calibration & Measurement/Write and Read Measurement  variable_name=Sensor_ID  variable_value=0  variable_type=uint8  numD=1  unitStr=""  descStr=""
      settings: AttributesFormatString=type:%<variable_type> Dimensions:%<numD>
  Bus Element Out2 : Outport  PortName=ID  Element=Sensor_IDst
  BusElementOut6 : Outport  PortName=ID  Element=Sensor_ID
  Bus Element Out : Outport  Port=2  PortName=Accel  Element=Sensor_Ast
  BusElementOut : Outport  Port=2  PortName=Accel  Element=Sensor_Ax
  BusElementOut1 : Outport  Port=2  PortName=Accel  Element=Sensor_Ay
  BusElementOut2 : Outport  Port=2  PortName=Accel  Element=Sensor_Az
  Bus Element Out1 : Outport  Port=3  PortName=Gyro  Element=Sensor_Gst
  BusElementOut3 : Outport  Port=3  PortName=Gyro  Element=Sensor_Gx
  BusElementOut4 : Outport  Port=3  PortName=Gyro  Element=Sensor_Gy
  BusElementOut5 : Outport  Port=3  PortName=Gyro  Element=Sensor_Gz
  Bus Element Out3 : Outport  Port=4  PortName=Temp  Element=Sensor_TempSt
  BusElementOut7 : Outport  Port=4  PortName=Temp  Element=Sensor_Temp
  wires:
  Read 6-Axis MEMS Sensor ID/1 -> Write and Read Measurement/1
  Read 6-Axis MEMS Sensor ID/2 -> Write and Read Measurement9/1
  Read Accel Data/1 -> Write and Read Measurement1/1
  Read Accel Data/2 -> Write and Read Measurement2/1
  Read Accel Data/3 -> Write and Read Measurement3/1
  Read Accel Data/4 -> Write and Read Measurement4/1
  Read Gyro Data/2 -> Write and Read Measurement6/1
  Read Gyro Data/3 -> Write and Read Measurement7/1
  Read Gyro Data/4 -> Write and Read Measurement8/1
  Read Gyro Data/1 -> Write and Read Measurement5/1
  Read Temperature/1 -> Write and Read Measurement10/1
  Read Temperature/2 -> Write and Read Measurement11/1
  Write and Read Measurement2/1 -> BusElementOut/1  "Sensor_Ax"
  Write and Read Measurement1/1 -> Bus Element Out/1  "Sensor_Ast"
  Write and Read Measurement3/1 -> BusElementOut1/1  "Sensor_Ay"
  Write and Read Measurement4/1 -> BusElementOut2/1  "Sensor_Az"
  Write and Read Measurement5/1 -> Bus Element Out1/1  "Sensor_Gst"
  Write and Read Measurement6/1 -> BusElementOut3/1  "Sensor_Gx"
  Write and Read Measurement7/1 -> BusElementOut4/1  "Sensor_Gy"
  Write and Read Measurement8/1 -> BusElementOut5/1  "Sensor_Gz"
  Write and Read Measurement/1 -> Bus Element Out2/1  "Sensor_IDst"
  Write and Read Measurement9/1 -> BusElementOut6/1  "Sensor_ID"
  Write and Read Measurement10/1 -> Bus Element Out3/1  "Sensor_TempSt"
  Write and Read Measurement11/1 -> BusElementOut7/1  "Sensor_Temp"

== system VHF_central_unit/ASW_Demo/01  process input signals/01 process electrical supply input signals/02 process electrical supply input signals/01 process battery voltage ==
  ADC Value To Volt : CoderSF_ADC2Volt_Libs/ADC Value To Volt  ResValue=12  RefValue=5  TypeOut=Inherit: Inherit via back propagation  WithDiv=on  DivValue=6.8  SerValue=15
  Read ADC Value : CoderSF_BSW_Libs/ADC/Read ADC Value  channel=28
  ecocoder_measurement1 : CoderSF_BSW_Libs/Calibration & Measurement/Write and Read Measurement  variable_name=sigInEsmBatt_volt  variable_value=0  variable_type=single  numD=1  unitStr=V  descStr=""
      settings: AttributesFormatString=value:%<variable_value> type:%<variable_type>
  sigInEsmBatt_volt : Outport
  wires:
  ADC Value To Volt/1 -> ecocoder_measurement1/1
  ecocoder_measurement1/1 -> sigInEsmBatt_volt/1  "sigInEsmBatt_volt"
  Read ADC Value/1 -> ADC Value To Volt/1

== system VHF_central_unit/ASW_Demo/01  process input signals/02 process driver input signals/01 link driver input signals/01 link key position ==
  LogicNOT1 : Logic  Operator=NOT  Inputs=1  AllPortsSameDT=off  OutDataTypeStr=boolean
  Switch Input : CoderSF_BSW_Libs/Digital I//O/Switch Input  portNum=DI_KEYON
  ecocoder_calibration : CoderSF_BSW_Libs/Calibration & Measurement/Read Calibration  variable_name=sigInLinkDrvKeyOn_flgPol_val  variable_value=0  variable_type=single  variable_min=[]  variable_max=[]  unitStr=""  descStr=""
      settings: AttributesFormatString=value:%<variable_value> type:%<variable_type> max:%<variable_max> Min:%<variable_min>
  ecocoder_measurement1 : CoderSF_BSW_Libs/Calibration & Measurement/Write and Read Measurement  variable_name=sigInLinkDrvKeyOn_flgEn  variable_value=0  variable_type=boolean  numD=1  unitStr=""  descStr=""
      settings: AttributesFormatString=value:%<variable_value> type:%<variable_type>
  if_then_else : EV_ASWLibs/if_then_else
  sigInLinkDrvKey_flgOn : Outport
  wires:
  ecocoder_calibration/1 -> if_then_else/1
  LogicNOT1/1 -> if_then_else/2
  Switch Input/1 -> LogicNOT1/1, if_then_else/3
  if_then_else/1 -> ecocoder_measurement1/1
  ecocoder_measurement1/1 -> sigInLinkDrvKey_flgOn/1  "sigInLinkDrvKeyOn_flgEn"

== system VHF_central_unit/ASW_Demo/01  process input signals/02 process driver input signals/01 link driver input signals/03 link accelerator pedal ==
  ADC Value To Volt : CoderSF_ADC2Volt_Libs/ADC Value To Volt  ResValue=12  RefValue=5  TypeOut=Inherit: Inherit via back propagation  WithDiv=off  DivValue=6.8  SerValue=15
  ADC Value To Volt1 : CoderSF_ADC2Volt_Libs/ADC Value To Volt  ResValue=12  RefValue=5  TypeOut=Inherit: Inherit via back propagation  WithDiv=off  DivValue=6.8  SerValue=15
  Read ADC Value : CoderSF_BSW_Libs/ADC/Read ADC Value  channel=39
  Read ADC Value1 : CoderSF_BSW_Libs/ADC/Read ADC Value  channel=37
  ecocoder_measurement1 : CoderSF_BSW_Libs/Calibration & Measurement/Write and Read Measurement  variable_name=sigInLinkDrvPedacc1_volt  variable_value=0  variable_type=single  numD=1  unitStr=V  descStr=""
      settings: AttributesFormatString=value:%<variable_value> type:%<variable_type>
  ecocoder_measurement2 : CoderSF_BSW_Libs/Calibration & Measurement/Write and Read Measurement  variable_name=sigInLinkDrvPedacc2_volt  variable_value=0  variable_type=single  numD=1  unitStr=V  descStr=""
      settings: AttributesFormatString=value:%<variable_value> type:%<variable_type>
  sigInLinkDrvPedacc_volt1 : Outport
  sigInLinkDrvPedacc_volt2 : Outport  Port=2
  wires:
  ADC Value To Volt/1 -> ecocoder_measurement1/1
  ADC Value To Volt1/1 -> ecocoder_measurement2/1
  ecocoder_measurement1/1 -> sigInLinkDrvPedacc_volt1/1  "sigInLinkDrvPedacc1_volt"
  ecocoder_measurement2/1 -> sigInLinkDrvPedacc_volt2/1  "sigInLinkDrvPedacc2_volt"
  Read ADC Value/1 -> ADC Value To Volt/1
  Read ADC Value1/1 -> ADC Value To Volt1/1

== system VHF_central_unit/ASW_Demo/01  process input signals/02 process driver input signals/02 process driver input signals/03 processs accelerator pedal ==
  sigInLinkDrvPedacc_volt1 : Inport
  sigInLinkDrvPedacc_volt2 : Inport  Port=2
  01 process accelerator pedal error : Subsystem  TreatAsAtomicUnit=on
      settings: RTWFcnNameOpts=Use subsystem name
  02 voltage selection : Subsystem  TreatAsAtomicUnit=on
      settings: RTWFcnNameOpts=Use subsystem name
  03 convert voltage to percentage : Subsystem  TreatAsAtomicUnit=on
      settings: RTWFcnNameOpts=Use subsystem name
  04 check plausibility : Subsystem  TreatAsAtomicUnit=on
      settings: RTWFcnNameOpts=Use subsystem name
  Constant : Constant  Value=false
  Constant1 : Constant  Value=false
  Terminator : Terminator
  sigInDrvPedacc_pct : Outport
  wires:
  04 check plausibility/1(sigInDrvPedacc_flgErrSync) -> Terminator/1
  [sigInDrvPedacc_volt2] -> 04 check plausibility/2(sigInDrvPedacc_volt2)
  [sigInDrvPedacc_volt1] -> 04 check plausibility/1(sigInDrvPedacc_volt1)
  02 voltage selection/2(sigInDrvPedacc_volt) -> 03 convert voltage to percentage/2(sigInDrvPedacc_volt)
  02 voltage selection/1(sigInDrvPedacc_stSigSrc) -> 03 convert voltage to percentage/1(sigInDrvPedacc_stSigSrc)
  Constant1/1 -> 02 voltage selection/3(diagDrvPedacc1_flgShrtPwr), 02 voltage selection/4(diagDrvPedacc2_flgShrtPwr), 02 voltage selection/5(diagDrvPedacc1_flgFinalDef), 02 voltage selection/6(diagDrvPedacc2_flgFinalDef), 02 voltage selection/7(diagDrvPedacc1_flgProvDef), 02 voltage selection/9(diagDrvPedacc2_flgProvDef), 02 voltage selection/10(diagDrvPedacc_flgSyncProvDef), 02 voltage selection/8(diagDrvPedacc_flgSyncDef)
  01 process accelerator pedal error/2(sigInDrvPedacc_volt2) -> [sigInDrvPedacc_volt2], 02 voltage selection/2(sigInDrvPedacc_volt2)
  01 process accelerator pedal error/1(sigInDrvPedacc_volt1) -> 02 voltage selection/1(sigInDrvPedacc_volt1), [sigInDrvPedacc_volt1]
  Constant/1 -> 01 process accelerator pedal error/3(diagDrvPedacc1_flgFinalDef), 01 process accelerator pedal error/4(diagDrvPedacc1_flgProvDef), 01 process accelerator pedal error/5(diagDrvPedacc2_flgFinalDef), 01 process accelerator pedal error/6(diagDrvPedacc2_flgProvDef)
  03 convert voltage to percentage/1(sigInDrvPedacc_pctFlt) -> sigInDrvPedacc_pct/1
  sigInLinkDrvPedacc_volt2/1 -> 01 process accelerator pedal error/2(sigInLinkDrvPedacc_volt2)
  sigInLinkDrvPedacc_volt1/1 -> 01 process accelerator pedal error/1(sigInLinkDrvPedacc_volt1)

== system VHF_central_unit/ASW_Demo/01  process input signals/03 process bms input signals/00 process bms input signals/02 process bms soc ==
  sigInBms_socRaw : Inport
  sigInBms_flgSocRawValid : Inport  Port=2
  DT_conv1 : DataTypeConversion  SaturateOnIntegerOverflow=off  RndMeth=Floor
  Switch : Switch  Criteria=u2 ~= 0  OutDataTypeStr=Inherit: Inherit via back propagation  SaturateOnIntegerOverflow=off
  ecocoder_measurement : CoderSF_BSW_Libs/Calibration & Measurement/Write and Read Measurement  variable_name=sigInBms_soc  variable_value=0  variable_type=single  numD=1  unitStr=%  descStr=""
      settings: AttributesFormatString=value:%<variable_value> type:%<variable_type>
  invalid ess soc output : Constant  Value=C_SOC_ZERO
      settings: AttributesFormatString=%<Value>\n%<OutDataTypeMode>
  sigInBms_soc : Outport
  wires:
  DT_conv1/1 -> Switch/1
  sigInBms_flgSocRawValid/1 -> Switch/2
  Switch/1 -> ecocoder_measurement/1
  sigInBms_socRaw/1 -> DT_conv1/1
  invalid ess soc output/1 -> Switch/3
  ecocoder_measurement/1 -> sigInBms_soc/1  "sigInBms_soc"

== system VHF_central_unit/ASW_Demo/01  process input signals/04 process traction motor input signals/00 process traction motor input signals/02 motor speed calculation ==
  sigInMot_rotspdRpm : Inport
  sigInMot_flgRotspdRpmValid : Inport  Port=2
  Switch : Switch  Criteria=u2 ~= 0  OutDataTypeStr=Inherit: Inherit via back propagation  SaturateOnIntegerOverflow=off
  ecocoder_measurement : CoderSF_BSW_Libs/Calibration & Measurement/Write and Read Measurement  variable_name=sigInTm_rotspd  variable_value=0  variable_type=single  numD=1  unitStr=rpm  descStr=""
      settings: AttributesFormatString=value:%<variable_value> type:%<variable_type>
  invalid motor speed output : Constant  Value=C_ROTSPD_ZERO
  sigInTm_rotspd : Outport
  wires:
  Switch/1 -> ecocoder_measurement/1
  sigInMot_rotspdRpm/1 -> Switch/1
  sigInMot_flgRotspdRpmValid/1 -> Switch/2
  invalid motor speed output/1 -> Switch/3
  ecocoder_measurement/1 -> sigInTm_rotspd/1  "sigInTm_rotspd"

== system VHF_central_unit/ASW_Demo/04 powertrain control /02  Bms control/02  Bms control/bmsc ==
  pwrtrn_st_i : Inport
  f : TriggerPort  TriggerType=function-call  VariantControl=(inherit)
  Constant : Constant  OutDataTypeStr=Inherit: Inherit via back propagation
  Terminator : Terminator
  pwrtrnBmscPack_flgConnReq : Outport
  wires:
  Constant/1 -> pwrtrnBmscPack_flgConnReq/1  "pwrtrnBmscPack_flgConnReq"
  pwrtrn_st_i/1 -> Terminator/1

== system VHF_central_unit/ASW_Demo/04 powertrain control /03  traction motor control/tmc/02 torque calculation ==
  vehDrv_trqReq : Inport
  pwrtrnTml_ratioShaftRotspd : Inport  Port=2
  sigInTm_rotspd : Inport  Port=3
  Data Type Conversion : DataTypeConversion  SaturateOnIntegerOverflow=off  RndMeth=Floor
  Divide : Product  Inputs=*/
  ecocoder_measurement : CoderSF_BSW_Libs/Calibration & Measurement/Write and Read Measurement  variable_name=pwrtrnTmc_trqReq  variable_value=0  variable_type=single  numD=1  unitStr=Nm  descStr=""
      settings: AttributesFormatString=value:%<variable_value> type:%<variable_type>
  terminator1 : Terminator
  pwrtrnTmc_trqReq : Outport
  wires:
  Data Type Conversion/1 -> Divide/2
  pwrtrnTml_ratioShaftRotspd/1 -> Data Type Conversion/1
  vehDrv_trqReq/1 -> Divide/1
  sigInTm_rotspd/1 -> terminator1/1
  Divide/1 -> ecocoder_measurement/1
  ecocoder_measurement/1 -> pwrtrnTmc_trqReq/1  "pwrtrnTmc_trqReq"

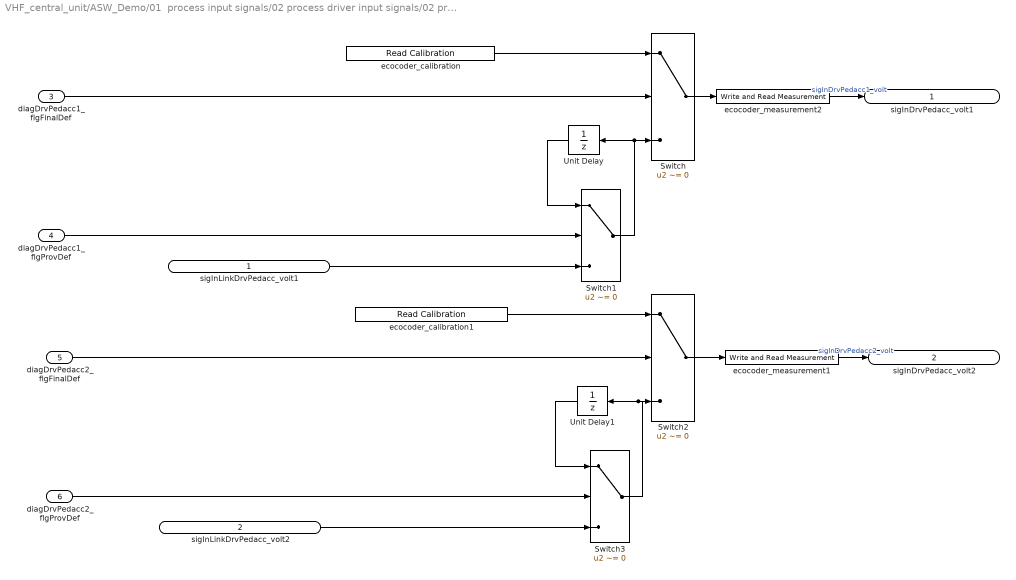
== system VHF_central_unit/ASW_Demo/01  process input signals/02 process driver input signals/02 process driver input signals/03 processs accelerator pedal/01 process accelerator pedal error ==
  sigInLinkDrvPedacc_volt1 : Inport
  sigInLinkDrvPedacc_volt2 : Inport  Port=2
  diagDrvPedacc1_flgFinalDef : Inport  Port=3
  diagDrvPedacc1_flgProvDef : Inport  Port=4
  diagDrvPedacc2_flgFinalDef : Inport  Port=5
  diagDrvPedacc2_flgProvDef : Inport  Port=6
  Switch{,1..3} (4 alike) : Switch  Criteria=u2 ~= 0  SaturateOnIntegerOverflow=off  InputSameDT=off
  Unit Delay : UnitDelay  SampleTime=-1
  Unit Delay1 : UnitDelay  SampleTime=-1
  ecocoder_calibration : CoderSF_BSW_Libs/Calibration & Measurement/Read Calibration  variable_name=sigInDrvPedacc1_voltDef_val  variable_value=0  variable_type=single  variable_min=[]  variable_max=[]  unitStr=V  descStr=""
      settings: AttributesFormatString=value:%<variable_value> type:%<variable_type> max:%<variable_max> Min:%<variable_min>
  ecocoder_calibration1 : CoderSF_BSW_Libs/Calibration & Measurement/Read Calibration  variable_name=sigInDrvPedacc1_voltDef_val  variable_value=0  variable_type=single  variable_min=[]  variable_max=[]  unitStr=V  descStr=""
      settings: AttributesFormatString=value:%<variable_value> type:%<variable_type> max:%<variable_max> Min:%<variable_min>
  ecocoder_measurement1 : CoderSF_BSW_Libs/Calibration & Measurement/Write and Read Measurement  variable_name=sigInDrvPedacc2_volt  variable_value=0  variable_type=single  numD=1  unitStr=V  descStr=""
      settings: AttributesFormatString=value:%<variable_value> type:%<variable_type>
  ecocoder_measurement2 : CoderSF_BSW_Libs/Calibration & Measurement/Write and Read Measurement  variable_name=sigInDrvPedacc1_volt  variable_value=0  variable_type=single  numD=1  unitStr=V  descStr=""
      settings: AttributesFormatString=value:%<variable_value> type:%<variable_type>
  sigInDrvPedacc_volt1 : Outport
  sigInDrvPedacc_volt2 : Outport  Port=2
  wires:
  Switch2/1 -> ecocoder_measurement1/1
  ecocoder_calibration1/1 -> Switch2/1
  diagDrvPedacc2_flgFinalDef/1 -> Switch2/2
  sigInLinkDrvPedacc_volt2/1 -> Switch3/3
  Switch3/1 -> Unit Delay1/1, Switch2/3
  Unit Delay1/1 -> Switch3/1
  diagDrvPedacc2_flgProvDef/1 -> Switch3/2
  Switch/1 -> ecocoder_measurement2/1
  ecocoder_calibration/1 -> Switch/1
  diagDrvPedacc1_flgFinalDef/1 -> Switch/2
  sigInLinkDrvPedacc_volt1/1 -> Switch1/3
  Switch1/1 -> Switch/3, Unit Delay/1
  Unit Delay/1 -> Switch1/1
  diagDrvPedacc1_flgProvDef/1 -> Switch1/2
  ecocoder_measurement2/1 -> sigInDrvPedacc_volt1/1  "sigInDrvPedacc1_volt"
  ecocoder_measurement1/1 -> sigInDrvPedacc_volt2/1  "sigInDrvPedacc2_volt"

== system VHF_central_unit/ASW_Demo/01  process input signals/02 process driver input signals/02 process driver input signals/03 processs accelerator pedal/02 voltage selection ==
  sigInDrvPedacc_volt1 : Inport
  sigInDrvPedacc_volt2 : Inport  Port=2
  diagDrvPedacc1_flgShrtPwr : Inport  Port=3
  diagDrvPedacc2_flgShrtPwr : Inport  Port=4
  diagDrvPedacc1_flgFinalDef : Inport  Port=5
  diagDrvPedacc2_flgFinalDef : Inport  Port=6
  diagDrvPedacc1_flgProvDef : Inport  Port=7
  diagDrvPedacc_flgSyncDef : Inport  Port=8
  diagDrvPedacc2_flgProvDef : Inport  Port=9
  diagDrvPedacc_flgSyncProvDef : Inport  Port=10
  SelSig_GetStSigSrc : Subsystem  TreatAsAtomicUnit=on
      settings: RTWSystemCode=Nonreusable function  RTWFcnNameOpts=Use subsystem name
  SelSig_GetURaw : Subsystem  TreatAsAtomicUnit=on
      settings: RTWSystemCode=Nonreusable function  RTWFcnNameOpts=Use subsystem name
  sigInDrvPedacc_stSigSrc : Outport
  sigInDrvPedacc_volt : Outport  Port=2
  wires:
  diagDrvPedacc2_flgProvDef/1 -> SelSig_GetURaw/6(diagDrvPedacc2_flgProvDef)
  diagDrvPedacc2_flgFinalDef/1 -> SelSig_GetStSigSrc/4(diagDrvPedacc2_flgFinalDef), SelSig_GetURaw/7(diagDrvPedacc2_flgFinalDef)
  diagDrvPedacc1_flgFinalDef/1 -> SelSig_GetStSigSrc/3(diagDrvPedacc1_flgFinalDef), SelSig_GetURaw/5(diagDrvPedacc1_flgFinalDef)
  diagDrvPedacc2_flgShrtPwr/1 -> SelSig_GetStSigSrc/2(diagDrvPedacc2_flgShrtPwr)
  diagDrvPedacc1_flgShrtPwr/1 -> SelSig_GetStSigSrc/1(diagDrvPedacc1_flgShrtPwr)
  diagDrvPedacc_flgSyncProvDef/1 -> SelSig_GetURaw/9(diagDrvPedacc_flgSyncProvDef)
  sigInDrvPedacc_volt2/1 -> SelSig_GetURaw/2(sigInDrvPedacc_volt2)
  sigInDrvPedacc_volt1/1 -> SelSig_GetURaw/3(sigInDrvPedacc_volt1)
  SelSig_GetURaw/1(sigInDrvPedacc_volt) -> sigInDrvPedacc_volt/1
  diagDrvPedacc_flgSyncDef/1 -> SelSig_GetURaw/8(diagDrvPedacc_flgSyncDef), SelSig_GetStSigSrc/5(diagDrvPedacc_flgSyncDef)
  diagDrvPedacc1_flgProvDef/1 -> SelSig_GetURaw/4(diagDrvPedacc1_flgProvDef)
  SelSig_GetStSigSrc/1(sigInDrvPedacc_stSigSrc) -> sigInDrvPedacc_stSigSrc/1, SelSig_GetURaw/1(sigInDrvPedacc_stSigSrc)

== system VHF_central_unit/ASW_Demo/01  process input signals/02 process driver input signals/02 process driver input signals/03 processs accelerator pedal/03 convert voltage to percentage ==
  sigInDrvPedacc_stSigSrc : Inport
  sigInDrvPedacc_volt : Inport  Port=2
  GetRUnFlt : Subsystem  TreatAsAtomicUnit=on
      settings: RTWSystemCode=Nonreusable function  RTWFcnNameOpts=Use subsystem name
  LPT_xxxx : EV_ASWLibs/LPT_xxxx
  Switch1 : Switch  Criteria=u2 ~= 0  RndMeth=Simplest  InputSameDT=off
  Terminator : Terminator
  ecocoder_calibration : CoderSF_BSW_Libs/Calibration & Measurement/Read Calibration  variable_name=sigInDrvPedacc_tFltPT1_val  variable_value=0  variable_type=single  variable_min=[]  variable_max=[]  unitStr=s  descStr=""
      settings: AttributesFormatString=value:%<variable_value> type:%<variable_type> max:%<variable_max> Min:%<variable_min>
  ecocoder_measurement : CoderSF_BSW_Libs/Calibration & Measurement/Write and Read Measurement  variable_name=sigInDrvPedacc_pct  variable_value=0  variable_type=single  numD=1  unitStr=""  descStr=""
      settings: AttributesFormatString=value:%<variable_value> type:%<variable_type>
  sigInDrvPedacc_pctFlt : Outport
  wires:
  Switch1/1 -> ecocoder_measurement/1
  sigInDrvPedacc_stSigSrc/1 -> Switch1/2
  sigInDrvPedacc_volt/1 -> GetRUnFlt/1(sigInDrvPedacc_volt)
  GetRUnFlt/1(sigInDrvPedacc_dpctUnFlt) -> Terminator/1
  GetRUnFlt/2(sigInDrvPedacc_pctUnFlt) -> Switch1/1, LPT_xxxx/2
  ecocoder_calibration/1 -> LPT_xxxx/1
  LPT_xxxx/1 -> Switch1/3
  ecocoder_measurement/1 -> sigInDrvPedacc_pctFlt/1  "sigInDrvPedacc_pct"

== system VHF_central_unit/ASW_Demo/01  process input signals/02 process driver input signals/02 process driver input signals/03 processs accelerator pedal/04 check plausibility ==
  sigInDrvPedacc_volt1 : Inport
  sigInDrvPedacc_volt2 : Inport  Port=2
  Constant : Constant  OutDataTypeStr=Inherit: Inherit via back propagation
  Terminator : Terminator
  Terminator1 : Terminator
  sigInDrvPedacc_flgErrSync : Outport
  wires:
  sigInDrvPedacc_volt1/1 -> Terminator/1
  Constant/1 -> sigInDrvPedacc_flgErrSync/1  "sigInDrvPedacc_flgErrSync"
  sigInDrvPedacc_volt2/1 -> Terminator1/1
